simulink model "MotorCoupledIdent"  (R2013a)
settings: Solver=FixedStepDiscrete  StartTime=0.0  StopTime=Time  FixedStep=0.01  RelTol=1e-3
values from neighbouring files (symbols this model uses):
  joint_number = [joint(1).number joint(2).number joint(3).number]    [CoupledJoints.m]
  joint_path = type    [CoupledJoints.m]
  Reference = struct    [CoupledJoints.m]    (also in ReferenceLoad.m; WBLMotor.m)
libraries: WBCLibrary x7, utility x1
settings Model: Creator=Raffaello  LastModifiedBy=Raffaello
settings DataIOCC: LimitDataPoints=off  OutputSaveName=out

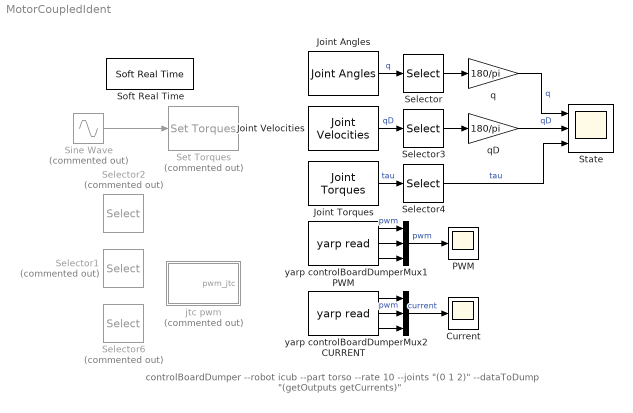
== system MotorCoupledIdent ==
  note: controlBoardDumper --robot icub --part torso --rate 10 --joints "(0 1 2)" --dataToDump "(getOutputs getCurrents)"
  Current : Scope
      settings: YMin=-3750  YMax=1750  SaveName=ScopeData2
  Joint Angles : WBCLibrary/wholeBodyStates/Joint Angles  robotName=robotName  localName=localName
  Joint Torques : WBCLibrary/wholeBodyStates/Joint Torques  robotName=robotName  localName=localName
  Joint Velocities : WBCLibrary/wholeBodyStates/Joint Velocities  robotName=robotName  localName=localName
  Mux1 : Mux  Inputs=3
  Mux2 : Mux  Inputs=3
  PWM : Scope
      settings: TimeRange=60  YMin=-60  YMax=60
  Selector : Selector  InputPortWidth=25  IndexOptions=Index vector (dialog)  Indices=[joint_number]  OutputSizes=1
  Selector1 : Selector  Commented=on  InputPortWidth=3  IndexOptions=Index vector (dialog)  Indices=[3 2 1]  OutputSizes=1
  Selector2 : Selector  Commented=on  InputPortWidth=3  IndexOptions=Index vector (dialog)  Indices=[3 2 1]  OutputSizes=1
  Selector3 : Selector  InputPortWidth=25  IndexOptions=Index vector (dialog)  Indices=[joint_number]  OutputSizes=1
  Selector4 : Selector  InputPortWidth=25  IndexOptions=Index vector (dialog)  Indices=[joint_number]  OutputSizes=1
  Selector6 : Selector  Commented=on  InputPortWidth=3  IndexOptions=Index vector (dialog)  Indices=[3 2 1]  OutputSizes=1
  Set Torques : WBCLibrary/wholeBodyActuators/Set Torques  Commented=on  val=6  robotName=robotName  localName=localName
  Sine Wave : Sin  Commented=on  Amplitude=Reference.sinAmp  Bias=Reference.sinBias  Frequency=Reference.sinFreq*2*pi  SampleTime=0
  Soft Real Time : utility/Soft Real Time  x=1
  State : Scope  NumInputPorts=3
      settings: TimeRange=60  YMin=-40~-10~-2.75  YMax=40~20~1.25  SaveName=ScopeData3
  jtc pwm : Subsystem  Commented=on
  q : Gain  Gain=180/pi
  qD : Gain  Gain=180/pi
  yarp controlBoardDumper CURRENT : WBCLibrary/Utilities/yarp read  from=['/controlBoardDumper/' joint_path '/getCurrents']  to='...'  num=3  blocking=off  timestamp=off
  yarp controlBoardDumper PWM : WBCLibrary/Utilities/yarp read  from=['/controlBoardDumper/' joint_path '/getOutputs']  to='...'  num=3  blocking=off  timestamp=off
  wires:
  Sine Wave/1 -> Set Torques/1
  Joint Angles/1 -> Selector/1  "q"
  Joint Velocities/1 -> Selector3/1  "qD"
  q/1 -> State/1  "q"
  qD/1 -> State/2  "qD"
  yarp controlBoardDumper PWM/1 -> Mux1/1  "pwm"
  yarp controlBoardDumper PWM/2 -> Mux1/2
  yarp controlBoardDumper PWM/3 -> Mux1/3
  Mux1/1 -> PWM/1  "pwm"
  yarp controlBoardDumper CURRENT/1 -> Mux2/1  "pwm"
  yarp controlBoardDumper CURRENT/2 -> Mux2/2
  yarp controlBoardDumper CURRENT/3 -> Mux2/3
  Mux2/1 -> Current/1  "current"
  Joint Torques/1 -> Selector4/1  "tau"
  Selector/1 -> q/1
  Selector3/1 -> qD/1
  Selector4/1 -> State/3  "tau"

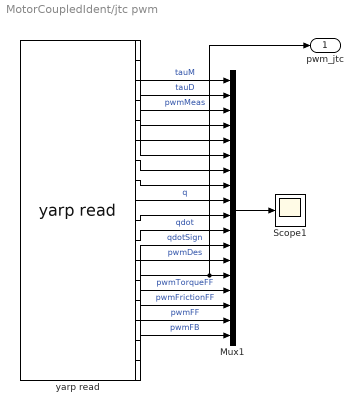
== system MotorCoupledIdent/jtc pwm ==
  Mux1 : Mux  Inputs=18
  Scope1 : Scope
      settings: ShowLegends=on
  yarp read : WBCLibrary/Utilities/yarp read  from=['/jtc/monitor:o']  to='...'  num=18  blocking=off  timestamp=off
  pwm_jtc : Outport
  wires:
  yarp read/18 -> Mux1/18  "pwmFB"
  Mux1/1 -> Scope1/1
  yarp read/1 -> Mux1/1  "tauM"
  yarp read/2 -> Mux1/2  "tauD"
  yarp read/3 -> Mux1/3
  yarp read/4 -> Mux1/4
  yarp read/5 -> Mux1/5
  yarp read/10 -> Mux1/10
  yarp read/6 -> Mux1/6
  yarp read/7 -> Mux1/7
  yarp read/8 -> Mux1/8
  yarp read/9 -> Mux1/9  "q"
  yarp read/11 -> Mux1/11  "qdot"
  yarp read/12 -> Mux1/12  "qdotSign"
  yarp read/13 -> Mux1/13  "pwmDes"
  yarp read/14 -> pwm_jtc/1, Mux1/14  "pwmMeas"
  yarp read/15 -> Mux1/15  "pwmTorqueFF"
  yarp read/16 -> Mux1/16  "pwmFrictionFF"
  yarp read/17 -> Mux1/17  "pwmFF"
